simulink model "line_tracking_algorithm_test_harness"  (R2013a)
settings: Solver=ode45  StartTime=0.0  StopTime=10.0  RelTol=1e-3
settings Model: Creator=mbiesiad  LastModifiedBy=mbiesiad
settings DataIOCC: SignalLoggingSaveFormat=ModelDataLogs
settings OptimizationCC: ExpressionDepthLimit=2147483647
settings DebuggingCC: MultiTaskDSMMsg=warning  MultiTaskCondExecSysMsg=none  StrictBusMsg=None
settings RTWCC: IncludeERTFirstTime=on

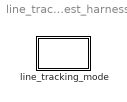
== system line_tracking_algorithm_test_harness ==
  line_tracking_mode : Stateflow chart  TreatAsAtomicUnit=on

== stateflow chart line_tracking_algorithm_test_harness/line_tracking_mode ==
  state line_tracking_mode
    during:
    current_mode_status = OperationModeStatusEnum.SUCCESSFULLY_COMPLETED;
  data: current_mode_status data_store_memory
